simulink model "equacao_diferencial"  (R2013a)
settings: Solver=ode45  StartTime=0.0  StopTime=10.0  RelTol=1e-3
settings Model: Creator=Felipe Bandeira  LastModifiedBy=Felipe Bandeira

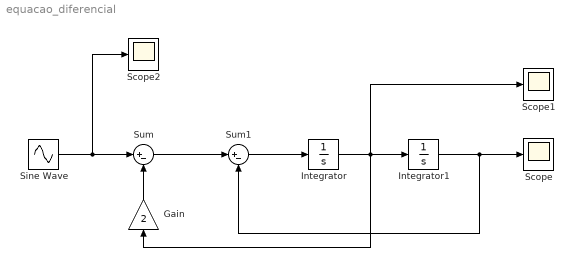
== system equacao_diferencial ==
  Gain : Gain  Gain=2
  Integrator : Integrator
  Integrator1 : Integrator
  Scope : Scope
  Scope1 : Scope
  Scope2 : Scope
      settings: SaveName=ScopeData2
  Sine Wave : Sin  Amplitude=10  Frequency=4  SampleTime=0
  Sum : Sum  Inputs=|+-
  Sum1 : Sum  Inputs=|+-
  wires:
  Sine Wave/1 -> Scope2/1, Sum/1
  Sum/1 -> Sum1/1
  Sum1/1 -> Integrator/1
  Integrator1/1 -> Sum1/2, Scope/1
  Integrator/1 -> Gain/1, Scope1/1, Integrator1/1
  Gain/1 -> Sum/2
